simulink model "SpearheadControlDesignSim"  (R2022b)
settings: Solver=VariableStepAuto  StartTime=0.0  StopTime=10.0  RelTol=1e-3
values from neighbouring files (symbols this model uses):
  adb = importdata('datafiles/mga_v2_adb.dat')    [adbCoefficientModel.m]    (also in spearheadAnalysis.m = importdata('datafiles/adb_w_hat.txt'); spearheadControl.m = importdata('spearheadData/ConfigurationData/adb_w_hat.txt'); spearheadControl2.m = importdata('spearheadData/ConfigurationData/adb_w_hat.txt'); spearheadCruiseAnalysis.m = importdata('spearheadData/ConfigurationData/adb_w_hat.txt'))
  l_elevon = importdata('datafiles/le_w_hat.txt')    [spearheadAnalysis.m]    (also in spearheadControl.m = importdata('spearheadData/ConfigurationData/le_w_hat.txt'); spearheadControl2.m = importdata('spearheadData/ConfigurationData/le_w_hat.txt'); surfaceCoefficientModel.m = importdata('datafiles/l_elevon.dat'))
  r_elevon = importdata('datafiles/re_w_hat.txt')    [spearheadAnalysis.m]    (also in spearheadControl.m = importdata('spearheadData/ConfigurationData/re_w_hat.txt'); spearheadControl2.m = importdata('spearheadData/ConfigurationData/re_w_hat.txt'); surfaceCoefficientModel.m = importdata('datafiles/r_elevon.dat'))
  rudder = importdata('datafiles/rudder_w_hat.txt')    [spearheadAnalysis.m]    (also in spearheadControl.m = importdata('spearheadData/ConfigurationData/rudder_w_hat.txt; spearheadControl2.m = importdata('spearheadData/ConfigurationData/rudder_w_hat.txt; surfaceCoefficientModel.m = importdata('datafiles/rudder.dat'))
  T = pascal(max(dim,deg))    [makepolymat.m]    (also in spearheadAnalysis.m = 0.01; spearheadControl.m = 0.001; spearheadControl2.m = 0.01; spearheadVerticalAnalysis.m = 0.01)
settings Model: Creator=alexd  LastModifiedBy=alexd

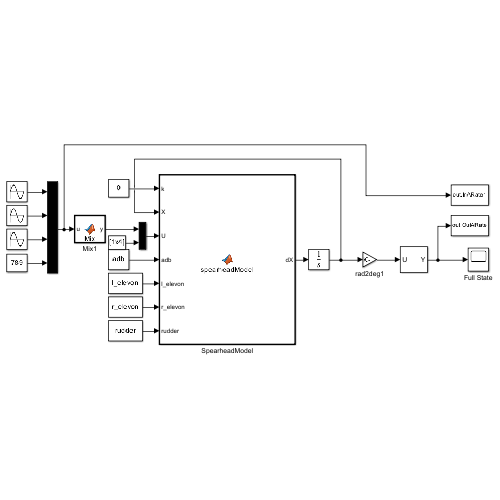
[thumbnail: Simulink's stored preview of the top-level diagram]
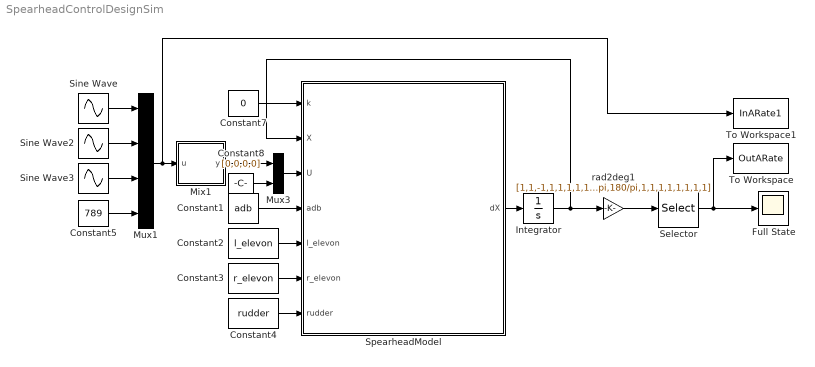
== system SpearheadControlDesignSim ==
  Constant1 : Constant  Value=adb  VectorParams1D=off
  Constant2 : Constant  Value=l_elevon  VectorParams1D=off
  Constant3 : Constant  Value=r_elevon  VectorParams1D=off
  Constant4 : Constant  Value=rudder  VectorParams1D=off
  Constant5 : Constant  Value=789
  Constant7 : Constant  Value=0
  Constant8 : Constant  Value=[0,0,0,0]
  Full State : Scope
  Integrator : Integrator  InitialCondition=[0;0;0;0;0;0;0;0;0;0;0;0;0;0;0;0;0;0;0;0]
  Mix1 : MATLAB Function  TreatAsAtomicUnit=on  SystemSampleTime=T
  Mux1 : Mux
  Mux3 : Mux  Inputs=2
  Selector : Selector  InputPortWidth=20  IndexOptions=Index vector (dialog)  Indices=[3,4,5,6]  OutputSizes=1
  Sine Wave : Sin  Frequency=60  SampleTime=0
  Sine Wave2 : Sin  Frequency=60  SampleTime=0
  Sine Wave3 : Sin  Frequency=60  SampleTime=0
  SpearheadModel : MATLAB Function  TreatAsAtomicUnit=on  SystemSampleTime=T
  To Workspace : ToWorkspace  VariableName=OutARate  SaveFormat=Timeseries  SampleTime=-1
  To Workspace1 : ToWorkspace  VariableName=InARate1  SaveFormat=Timeseries  SampleTime=-1
  rad2deg1 : Gain  Gain=[1,1,-1,1,1,1,1,1,-1,180/pi,180/pi,180/pi,1,1,1,1,1,1,1,1]  SaturateOnIntegerOverflow=on  OutDataTypeStr=Inherit: Same as input  ParamDataTypeStr=Inherit: Same as input
  wires:
  Constant7/1 -> SpearheadModel/1(k)
  SpearheadModel/1(dX) -> Integrator/1
  Constant4/1 -> SpearheadModel/7(rudder)
  Constant3/1 -> SpearheadModel/6(r_elevon)
  Constant2/1 -> SpearheadModel/5(l_elevon)
  Constant1/1 -> SpearheadModel/4(adb)
  Mux3/1 -> SpearheadModel/3(U)
  Constant8/1 -> Mux3/2
  Mix1/1(y) -> Mux3/1
  rad2deg1/1 -> Selector/1
  Integrator/1 -> SpearheadModel/2(X), rad2deg1/1
  Mux1/1 -> To Workspace1/1, Mix1/1(u)
  Sine Wave/1 -> Mux1/1
  Sine Wave2/1 -> Mux1/2
  Sine Wave3/1 -> Mux1/3
  Selector/1 -> To Workspace/1, Full State/1
  Constant5/1 -> Mux1/4

== matlab function SpearheadControlDesignSim/SpearheadModel ==
  data: k input; dX output; X input; U input; adb input; l_elevon input; r_elevon input; rudder input
function dX  = spearheadModel(k,X,U,adb,l_elevon,r_elevon,rudder)
%% Xdot = f(X,U)

%% Mass of the VTOL Craft as Taken From CAD
M = 20;
g = 9.81;
rho = 1.225; % sea level air density

%% VTOL Dimensions
% CG at [0.6, 0, 0] m.
L1 = 1.65;
L2 = 1.425;
C = 0.32; % Wing Mean Cord Length
S = 2.24; % Wing Planform Area
eS = 0.28*0.58;% Elevon Planform Area chord x span
rS = 0.32*0.30;% Rudder Planform Area chord x span

%% Mass Moment of Inertia about the COM As Taken From CAD
Ixx = 8.734;
Iyy = 5.592;
Izz = 13.623;

%% X = [u v w p q r x y z phi theta psi w1 w2 w3 w4 w5 dl dr drd]
% Linear and Angular Velocity in Fb (m/s and rads/s)
u = X(1);
v = X(2);
w = X(3);
p = X(4);
q = X(5);
r = X(6);
% Linear and Angular position in Fe (meters and rads)
x = X(7);
y = X(8);
z = X(9);
phi = X(10);
theta = X(11);
psi = X(12);
% Motor angular velocity (RPM)
w1 = X(13);
w2 = X(14);
w3 = X(15);
w4 = X(16);
w5 = X(17);
% Control Surface Defelection Angles(degrees)
dl = X(18);
dr = X(19);
drd = X(20);

%% U = [u1 u2 u3 u4 u5 u6 u7 u8] K = Motor Gain Mau = Time Constant Ku = Input Gain
K = [1.123*10^-6; 2.25*10^-6; 7.708*10^-7; 18.708*10^-7];
Mtau = [1/44.22; 1/44.22; 1/20];
Ku = [44.2205*8.18; 44.2205*7.02; 3.6];

F1 = K(1)*w1*w1;
F2 = K(1)*w2*w2;    
F3 = K(1)*w3*w3;
F4 = K(1)*w4*w4;

F5 = K(2)*w5*w5;

Tau1 = K(3)*w1*w1;
Tau2 = -K(3)*w2*w2;
Tau3 = -K(3)*w3*w3;
Tau4 = K(3)*w4*w4;

Tau5 = K(4)*w5*w5;

Fn = F1+F2+F3+F4;
Taun = Tau1+Tau2+Tau3+Tau4;

%% Wind Frame Variables: V = Airspeed alpha = AngleofAttack beta = AngleofSideslip
todeg = 180/pi;
V = sqrt(u*u + v*v + w*w);
alpha = atan2(w,u)*todeg;

if V == 0
  beta = 0;
else
  beta = asin(v/V)*todeg;
end

%% Aerodynamic Coefficients: ['CFX','CFY','CFZ','CMX','CMY','CMZ']
adb_C = adbCoefficients(alpha,beta,adb);
le_C = [1 dl dl^2 dl^3 dl^4 dl^5 dl^6 dl^7 dl^8]*l_elevon;
re_C = [1 dr dr^2 dr^3 dr^4 dr^5 dr^6 dr^7 dr^8]*r_elevon;
rudder_C = [1 drd drd^2 drd^3 drd^4 drd^5 drd^6 drd^7 drd^8]*rudder;

%% Forces: Thrust
FTx = F5;
FTy = 0;
FTz = -Fn;

%% Forces: Gravity
FGx = -g*sin(theta);
FGy = g*sin(phi)*cos(theta);
FGz = g*cos(phi)*cos(theta);

%% Forces: Aerodynamic [Drag,Sideforce,Lift]
FAx = 0.5 * rho * V*V * (S * adb_C(1) + eS * le_C(1) + eS * re_C(1) + rS * rudder_C(1));
FAy = 0.5 * rho * V*V * (S * adb_C(2) + eS * le_C(2) + eS * re_C(2) + rS * rudder_C(2));
FAz = 0.5 * rho * V*V * (S * adb_C(3) + eS * le_C(3) + eS * re_C(3) + rS * rudder_C(3));

%% Moments: Thrust
LT = L1*((F1 + F3) - (F2 + F4)) + Tau5;
MT = L2*((F1 + F2) - (F3 + F4));
NT = Taun;

%% Moments: Aerodynamic [Roll,Pitch,Yaw]
LA = 0.5 * rho * V*V * C * (S * adb_C(4) + eS * le_C(4) + eS * re_C(4) + rS * rudder_C(4));
MA = 0.5 * rho * V*V * C * (S * adb_C(5) + eS * le_C(5) + eS * re_C(5) + rS * rudder_C(5));
NA = 0.5 * rho * V*V * C * (S * adb_C(6) + eS * le_C(6) + eS * re_C(6) + rS * rudder_C(6));

%% 6-DOF Dynamics: dX = [udot vdot wdot pdot qdot rdot xdot ydot zdot phidot thetadot psidot]
dX1 = FGx + FAx/M + FTx/M - q*w + r*v;%# + g*sin(theta);
dX2 = FGy + FAy/M + FTy/M - r*u + p*w;
dX3 = FGz + FAz/M + FTz/M - p*v + q*u;%# - g*cos(theta);
dX4 = LA/Ixx + LT/Ixx - q*r*(Izz - Iyy)/Ixx;
dX5 = MA/Iyy + MT/Iyy - p*r*(Ixx - Izz)/Iyy;
dX6 = NA/Izz + NT/Izz - p*q*(Iyy - Ixx)/Izz;

dX7 = u*(cos(theta)*cos(psi)) + v*(sin(phi)*sin(theta)*cos(psi) - cos(phi)*sin(psi)) + w*(cos(phi)*sin(theta)*cos(psi) + sin(phi)*sin(psi));
dX8 = u*(cos(theta)*sin(psi)) + v*(sin(phi)*sin(theta)*sin(psi) + cos(phi)*cos(psi)) + w*(cos(phi)*sin(theta)*sin(psi) - sin(phi)*cos(psi));
dX9 = -u*(sin(theta)) + v*(sin(phi)*cos(theta)) + w*(cos(phi)*cos(theta));
dX10 = p + q*(sin(phi)*tan(theta)) + r*(cos(phi)*tan(theta));
dX11 = q*cos(phi) - r*sin(phi);
dX12 = q*(sin(phi)/cos(theta)) + r*(cos(phi)/cos(theta));

%% Motor Dynamics: dX = [w1dot w2dot w3dot w4dot w5dot], U = Pulse Width of the pwm signal 0-1000
dX13 = -(1/Mtau(1))*w1 + Ku(1)*U(1);
dX14 = -(1/Mtau(1))*w2 + Ku(1)*U(2);
dX15 = -(1/Mtau(1))*w3 + Ku(1)*U(3);
dX16 = -(1/Mtau(1))*w4 + Ku(1)*U(4);
dX17 = -(1/Mtau(2))*w5 + Ku(2)*U(5);

%% Servo Dynamics: dX = [w6dot w7dot w8dot], U = Pulse Width of the pwm signal 0-1000
dX18 = -(1/Mtau(3))*dl + Ku(3)*U(6);
dX19 = -(1/Mtau(3))*dr + Ku(3)*U(7);
dX20 = -(1/Mtau(3))*drd + Ku(3)*U(8);

dX = [dX1;dX2;dX3;dX4;dX5;dX6;dX7;dX8;dX9;dX10;dX11;dX12;dX13;dX14;dX15;dX16;dX17;dX18;dX19;dX20];
end

== matlab function SpearheadControlDesignSim/Mix1 ==
  data: u input; y output
function y = Mix(u)
M = 20;
L1 = 1.65;
L2 = 1.425;
Ixx = 5.061E+05;
Iyy = 5.061E+05;
Izz = 10.011E+05;
K = 1.123*10^-6;
K2 = 7.708*10^-7;
Ku = 44.2205*8.18;

%{
Usqr = [L1*K/Ixx, -L1*K/Ixx, L1*K/Ixx, -L1*K/Ixx;
        L2*K/Iyy, L2*K/Iyy, -L2*K/Iyy, -L2*K/Iyy;
        K2/Izz,    -K2/Izz,   -K2/Izz,    K2/Izz;
        -K/M,      -K/M,      -K/M,      -K/M]\u;
%}

Usqr = [(u(1) + u(2) + u(3) - u(4));
        (-u(1) + u(2) - u(3) - u(4));
        (u(1) - u(2) - u(3) - u(4));
        (-u(1) - u(2) + u(3) - u(4))];

%{
Usqr = [((L1/Ixx)*K*Ku*u(1) + (L2/Iyy)*K*Ku*u(2) + (1/Izz)*K2*Ku*u(3) - M*Ku*K*u(4));
        (-(L1/Ixx)*K*Ku*u(1) + (L2/Iyy)*K*Ku*u(2) - (1/Izz)*K2*Ku*u(3) - M*Ku*K*u(4));
        ((L1/Ixx)*K*Ku*u(1) - (L2/Iyy)*K*Ku*u(2) - (1/Izz)*K2*Ku*u(3) - M*Ku*K*u(4));
        (-(L1/Ixx)*K*Ku*u(1) - (L2/Iyy)*K*Ku*u(2) + (1/Izz)*K2*Ku*u(3) - M*Ku*K*u(4))];
%}
%y = sqrt(abs(Usqr))/Ku;

y = Usqr;
